simulink subsystem "MCU"  (R2023a)
settings: Solver=VariableStepAuto  StartTime=0.0  StopTime=10.0  RelTol=1e-3
model mask{kp=1, ki=1, kd=1, kn=kn}
  mask prompts: kp "коэфициент прямой связи ПИД регулятора"; ki "коэфициент интегральной связи ПИД регулятора"; kd "коэфициент дифференциальной связи ПИД регулятора"; kn "коэффициент усиления низкоуровнего контроллера"
settings Model: Creator=diontep  LastModifiedBy=diontep

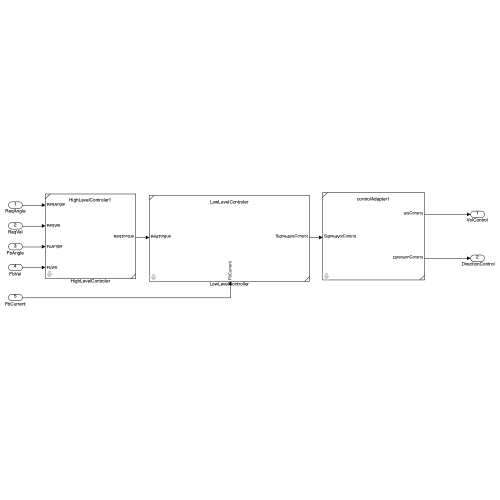
[thumbnail: Simulink's stored preview of the top-level diagram]
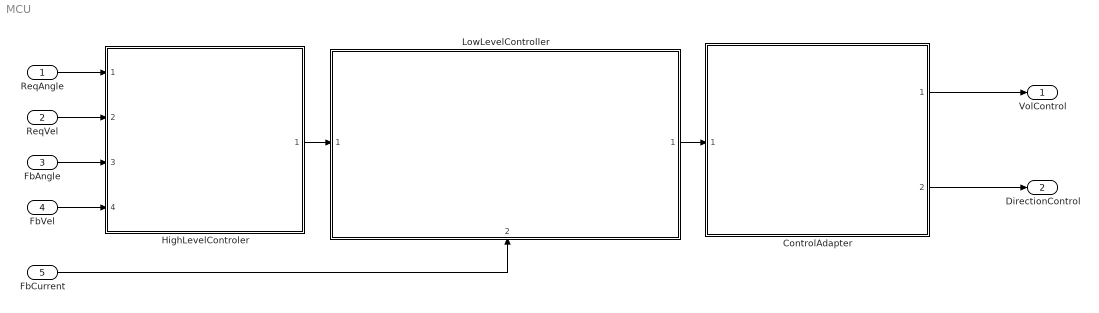
== system MCU ==
  ReqAngle : Inport
  ReqVel : Inport  Port=2
  FbAngle : Inport  Port=3
  FbVel : Inport  Port=4
  FbCurrent : Inport  Port=5
  ControlAdapter : Subsystem  ReferencedSubsystem=controlAdapter1
  HighLevelControler : Subsystem  ReferencedSubsystem=HighLevelControler1  kp=kp  ki=ki  kd=kd
  LowLevelController : Subsystem  ReferencedSubsystem=LowLevelControler  K_m=0.016  Gain=kn
      settings: PortSchema="{\"entries\":[{\"content\":{\"sides\":[{\"content\":{\"connectorIds\":[\"In1\"]},\"type\":\"ConnectorPlacement.EquallySpacedRectSide\",\"uuid\":\"8c9ae34d-fd19-467b-8264-bff91b0ebdf6\"},{\"content\":{\"connectorIds\":[\"Out1\"],\"side\":\"RIGHT\"},\"type\":\"ConnectorPlacement.EquallySpacedRectSide\",\"uuid\":\"dcf65e7e-3503-4c03-992a-e3cf270f0a96\"},{\"content\":{\"side\":\"TOP\"},\"type\":\"ConnectorPlacement.EquallySpacedRectSide\",\"uuid\":\"fbf6a28d-1403-428a-9782-f3b763c1034c\"},{\"content\":{\"connectorIds\":[\"In2\"],\"side\":\"BOTTOM\"},\"type\":\"ConnectorPlacement.EquallySpacedRectSide\",\"uuid\":\"8f469106-86f7-471b-9b49-9c7d87ce6d66\"}]},\"type\":\"ConnectorPlacement.EquallySpacedConnector\",\"uuid\":\"49c48951-4919-4403-ad4b-a9990de523e0\"}],\"packageUris\":[\"http://schema.mathworks.com/mf0/Connector/R2020b\"],\"version\":\"1.0\"}"
  VolControl : Outport
  " DirectionControl" : Outport  Port=2
  wires:
  FbVel/1 -> HighLevelControler/4
  HighLevelControler/1 -> LowLevelController/1
  FbAngle/1 -> HighLevelControler/3
  ReqVel/1 -> HighLevelControler/2
  LowLevelController/1 -> ControlAdapter/1
  FbCurrent/1 -> LowLevelController/2
  ReqAngle/1 -> HighLevelControler/1
  ControlAdapter/1 -> VolControl/1
  ControlAdapter/2 -> " DirectionControl"/1
